simulink model "time_domain_AFE_1"  (R2025b)
settings: Solver=ode1  StartTime=0.0  StopTime=simlength  FixedStep=ts_afe_1  RelTol=1e-3
undefined symbols (not defined in the file): omega_base, ts_afe_1
settings Model: Creator=ltnbda  LastModifiedBy=dbagn

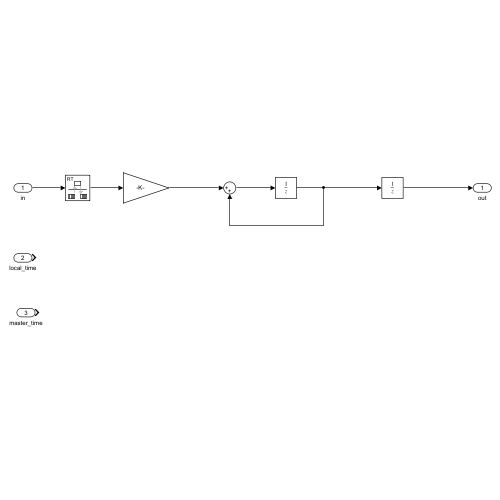
[thumbnail: Simulink's stored preview of the top-level diagram]
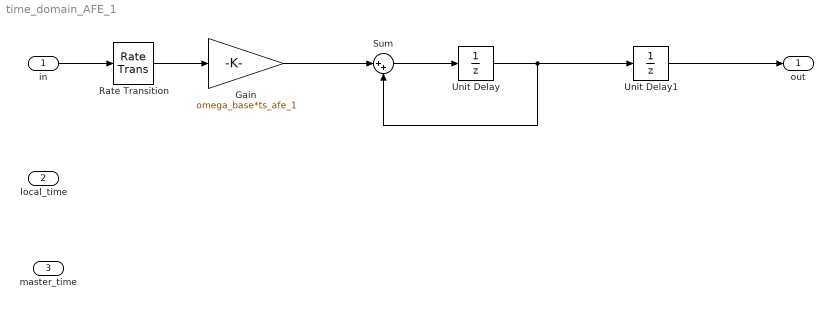
== system time_domain_AFE_1 ==
  in : Inport
  local_time : Inport  Port=2
  master_time : Inport  Port=3
  Gain : Gain  Gain=omega_base*ts_afe_1
  Rate Transition : RateTransition  OutPortSampleTime=ts_afe_1
  Sum : Sum  Inputs=|++
  Unit Delay : UnitDelay  SampleTime=ts_afe_1  HasFrameUpgradeWarning=on
  Unit Delay1 : UnitDelay  SampleTime=ts_afe_1  HasFrameUpgradeWarning=on
  out : Outport
  wires:
  Unit Delay/1 -> Sum/2, Unit Delay1/1
  Gain/1 -> Sum/1
  Sum/1 -> Unit Delay/1
  Unit Delay1/1 -> out/1
  in/1 -> Rate Transition/1
  Rate Transition/1 -> Gain/1
